simulink model "q2_5"  (R2018a)
settings: Solver=FixedStepDiscrete  StartTime=0.0  StopTime=2  FixedStep=0.000001  MaxStep=0.000001  RelTol=1e-3
libraries: powerlib x13
settings Model: Creator=MONSTER  LastModifiedBy=Berkay SAGLAM

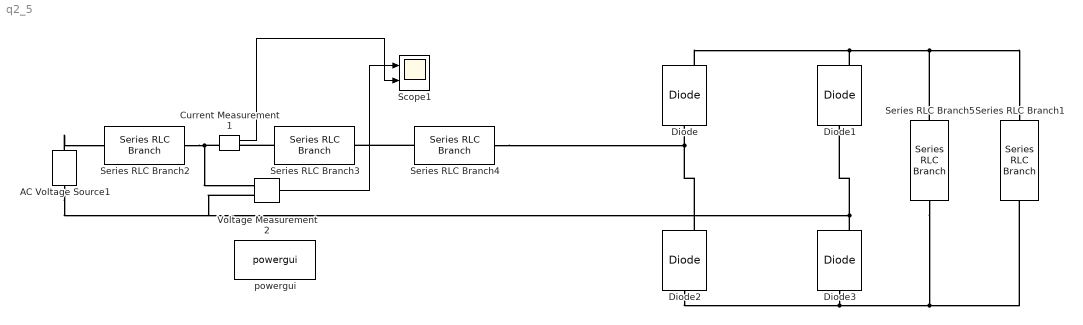
== system q2_5 ==
  AC Voltage Source1 : powerlib/Electrical Sources/AC Voltage Source  Amplitude=325.26912  Phase=0  Frequency=50  SampleTime=0  Measurements=Voltage  BusType=swing  Pref=10e3  Qref=0  Qmin=-inf  Qmax=+inf
  Current Measurement1 : powerlib/Measurements/Current Measurement  PhasorSimulation=off  OutputType=Complex  PSBequivalent=0
  Diode{,1..3} (4 alike) : powerlib/Power Electronics/Diode  Ron=0.001  Lon=0  Vf=0.8  IC=0  UseSnubber=0  Rs=500  Cs=250e-9  Measurements=on
  Scope1 : Scope  NumInputPorts=2
  Series RLC Branch1 : powerlib/Elements/Series RLC Branch  LConnTagsString=__new0  RConnTagsString=__new0  BranchType=R  Resistance=25  SetiL0=off  InitialCurrent=0  Setx0=off  InitialVoltage=0  Measurements=Branch voltage
      settings: AttributesFormatString=|
      | %<Resistance>
      | %<Inductance>
  Series RLC Branch2 : powerlib/Elements/Series RLC Branch  LConnTagsString=__new0  RConnTagsString=__new0  BranchType=L  Inductance=600e-6  SetiL0=off  InitialCurrent=0  Setx0=off  InitialVoltage=0  Measurements=Branch voltage
      settings: AttributesFormatString=|
      | %<Resistance>
      | %<Inductance>
  Series RLC Branch3 : powerlib/Elements/Series RLC Branch  LConnTagsString=__new0  RConnTagsString=__new0  BranchType=L  Inductance=600e-6  SetiL0=off  InitialCurrent=0  Setx0=off  InitialVoltage=0  Measurements=Branch voltage
      settings: AttributesFormatString=|
      | %<Resistance>
      | %<Inductance>
  Series RLC Branch4 : powerlib/Elements/Series RLC Branch  LConnTagsString=__new0  RConnTagsString=__new0  BranchType=R  Resistance=0.1  SetiL0=off  InitialCurrent=0  Setx0=off  InitialVoltage=0  Measurements=Branch voltage
      settings: AttributesFormatString=|
      | %<Resistance>
      | %<Inductance>
  Series RLC Branch5 : powerlib/Elements/Series RLC Branch  LConnTagsString=__new0  RConnTagsString=__new0  BranchType=C  SetiL0=off  InitialCurrent=0  Capacitance=2e-3  Setx0=off  InitialVoltage=0  Measurements=Branch voltage
      settings: AttributesFormatString=|
      | %<Resistance>
      | %<Inductance>
      | %<Capacitance>
  Voltage Measurement2 : powerlib/Measurements/Voltage Measurement  PhasorSimulation=off  OutputType=Complex  PSBequivalent=0
  powergui : powerlib/powergui  Priority=1  SimulationMode=Discrete  SampleTime=0.000001  frequency=60  Iterations=50  frequencyindice=50  Pbase=100e6  ErrMax=1e-4  UnitsV=kV  UnitsW=MW  buscounter=0  FunctionMessages=off  echomessages=off  EnableUseOfTLC=off  CurrentSourceSwitches=off  DisableSnubberDevices=off  DisableRonSwitches=off  DisableVfSwitches=off  DisplayEquations=off  SolverType=Tustin/Backward Euler (TBE)  Interpol=off  ExternalGateDelay=off  methode=off  Ts=100  x0status=blocks  SPID=off  SwTol=0  HookPort=off  RestoreLinks=warning  ResistiveCurrentMeasurement=off  Frange=[0:2:500]  Ylog=off  Xlog=on  ShowGrid=off  save=off  variable=ZData  structure=ScopeData1  ZoomFFT=off  StartTime=1.6  cycles=5  DisplayStyle=1  fundamental=50  FreqAxis=on  MaxFrequency=1000  frequencyindicesteady=1  RmsSteady=1  display=off
  wires:
  Current Measurement1/1 -> Scope1/2
  Voltage Measurement2/1 -> Scope1/1
  connections:
  Diode/RConn1 -- Diode1/RConn1 -- Series RLC Branch5/LConn1 -- Series RLC Branch1/LConn1
  Diode3/RConn1 -- Voltage Measurement2/LConn2 -- AC Voltage Source1/LConn1 -- Diode1/LConn1
  Diode2/RConn1 -- Series RLC Branch4/RConn1 -- Diode/LConn1
  Diode3/LConn1 -- Diode2/LConn1 -- Series RLC Branch5/RConn1 -- Series RLC Branch1/RConn1
  Current Measurement1/LConn1 -- Series RLC Branch2/RConn1 -- Voltage Measurement2/LConn1
  AC Voltage Source1/RConn1 -- Series RLC Branch2/LConn1
  Series RLC Branch3/LConn1 -- Current Measurement1/RConn1
  Series RLC Branch4/LConn1 -- Series RLC Branch3/RConn1
